simulink model "ControlSystemsLab_Peltier"  (R2017b)
settings: Solver=FixedStepDiscrete  StartTime=0.0  StopTime=10.0  FixedStep=1e-3  RelTol=1e-3
libraries: mbed_lib x9
settings Model: Creator=oh  LastModifiedBy=oh
settings DataIOCC: LimitDataPoints=on  SaveFormat=Array
settings OptimizationCC: DefaultParameterBehavior=Inlined  PassReuseOutputArgsAs=Individual arguments
settings DebuggingCC: SolverPrmCheckMsg=warning  ParameterTunabilityLossMsg=error  SFUnexpectedBacktrackingDiag=warning  SFNoUnconditionalDefaultTransitionDiag=warning  SFExecutionAtInitializationDiag=none
settings HardwareCC: ProdBitPerPointer=32  ProdBitPerSizeT=32  ProdBitPerPtrDiffT=32  ProdLargestAtomicInteger=Long  ProdLargestAtomicFloat=Double  ProdWordSize=32  ProdHWDeviceType=ARM Compatible->ARM Cortex
settings ModelReferenceCC: PropagateSignalLabelsOutOfModel=off
settings SFSimCC: MATLABDynamicMemAlloc=off
settings RTWCC: SystemTargetFile=mbed.tlc  TemplateMakefile=mbed.tmf  Description=MbedTarget (Embedded Target for Embedded Coder)  IncludeHyperlinkInReport=on  TargetLang=C++
settings CodeAppCC: ForceParamTrailComments=on  IgnoreCustomStorageClasses=off  OperatorAnnotations=on  SimulinkDataObjDesc=on  SFDataObjDesc=on  InsertBlockDesc=on
settings STFCustomTargetCC: TargetLibSuffix=.a  MultiwordLength=256  GenerateSampleERTMain=on  CombineOutputUpdateFcns=on  ERTCustomFileBanners=on  SupportContinuousTime=off  SupportNonInlinedSFcns=off  RemoveResetFunc=on  MATLABClassNameForMDSCustomization=Simulink.SoftwareTarget.ERTCustomization  ModelStepFunctionPrototypeControlCompliant=on  GRTInterface=off  SystemTargetFile=mbed.tlc
settings ERTTargetCC: GenerateSampleERTMain=on  ParMdlRefBuildCompliant=off  CompOptLevelCompliant=off  ConcurrentExecutionCompliant=off  CPPClassGenCompliant=off  UseToolchainInfoCompliant=off  InlinedParameterPlacement=NonHierarchical  ERTCustomFileTemplate=mbed_file_process.tlc
settings ConfigComp: CovMetricSettings=dw  CovHtmlReporting=on  CovSaveCumulativeToWorkspaceVar=on  CovSaveSingleToWorkspaceVar=on  CovExternalEMLEnable=off  CovSFcnEnable=off

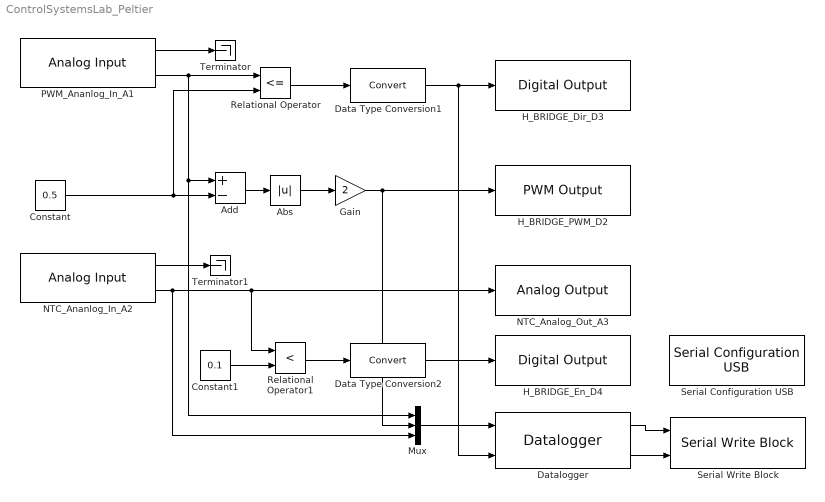
== system ControlSystemsLab_Peltier ==
  Abs : Abs
  Add : Sum  Inputs=+-
  Constant : Constant  Value=0.5  OutDataTypeStr=single
  Constant1 : Constant  Value=0.1  OutDataTypeStr=single
  Data Type Conversion1 : DataTypeConversion
  Data Type Conversion2 : DataTypeConversion
  Datalogger : mbed_lib/Utilities/Datalogger  TypeInputPorts={ 'single' 3 'uint8' 1 }  TypeOfInputs={'3*single' '1*uint8'}  BufferSize=100  errEn=off  SampleTime=-1
      settings: SourceProductName=Mbed Target
  Gain : Gain  Gain=2  OutDataTypeStr=single
  "H_BRIDGE_Dir_D3 " : mbed_lib/GPIO/Digital Output  PortName=B  PinNumber=0  OutputMode=PullDefault  SampleTime=-1
      settings: SourceProductName=Mbed Target
  H_BRIDGE_En_D4 : mbed_lib/GPIO/Digital Output  PortName=B  PinNumber=7  OutputMode=PullDefault  SampleTime=-1
      settings: SourceProductName=Mbed Target
  H_BRIDGE_PWM_D2 : mbed_lib/GPIO/PWM Output  PortName=A  PinNumber=12  Period=1000  SampleTime=-1
      settings: SourceProductName=Mbed Target
  Mux : Mux  Inputs=3
  NTC_Analog_Out_A3 : mbed_lib/GPIO/Analog Output  PortName=A  PinNumber=4  Mode=Double: 0 - 1.0f  SampleTime=-1
      settings: SourceProductName=Mbed Target
  NTC_Ananlog_In_A2 : mbed_lib/GPIO/Analog Input  PortName=A  PinNumber=3  SampleTime=0.001
      settings: SourceProductName=Mbed Target
  PWM_Ananlog_In_A1 : mbed_lib/GPIO/Analog Input  PortName=A  PinNumber=6  SampleTime=0.001
      settings: SourceProductName=Mbed Target
  Relational Operator : RelationalOperator  Operator=<=  RndMeth=Nearest
  Relational Operator1 : RelationalOperator  Operator=<  RndMeth=Nearest
  Serial Configuration USB : mbed_lib/Serial/UART/Serial Configuration USB  BaudRate=115200
      settings: SourceProductName=Mbed Target
  Serial Write Block : mbed_lib/Serial/UART/Serial Write Block  SerialPort=USB  numData=on  SampleTime=-1
      settings: SourceProductName=Mbed Target
  Terminator : Terminator
  Terminator1 : Terminator
  wires:
  Datalogger/1 -> Serial Write Block/1
  PWM_Ananlog_In_A1/2 -> Add/1, Mux/1, Relational Operator/1
  Constant/1 -> Relational Operator/2, Add/2
  Add/1 -> Abs/1
  Abs/1 -> Gain/1
  Gain/1 -> Mux/2, H_BRIDGE_PWM_D2/1
  Relational Operator/1 -> Data Type Conversion1/1
  Data Type Conversion1/1 -> Datalogger/2, "H_BRIDGE_Dir_D3 "/1
  NTC_Ananlog_In_A2/2 -> NTC_Analog_Out_A3/1, Relational Operator1/1, Mux/3
  Mux/1 -> Datalogger/1
  Constant1/1 -> Relational Operator1/2
  Relational Operator1/1 -> Data Type Conversion2/1
  Data Type Conversion2/1 -> H_BRIDGE_En_D4/1
  PWM_Ananlog_In_A1/1 -> Terminator/1
  NTC_Ananlog_In_A2/1 -> Terminator1/1
  Datalogger/2 -> Serial Write Block/2
